simulink model "QueuingStrategies_513"  (R2019b)
settings: Solver=VariableStepAuto  StartTime=0.0  StopTime=1000  RelTol=1e-3  EnableMultiTasking=on
InitFcn:
  | a = randi(600);
  | rng(a)
undefined symbols (not defined in the file or in its folder): elapsedTime, entity, m, n, whichLine
libraries: simulink x1
settings Model: Creator=The MathWorks, Inc.  LastModifiedBy=thb
settings DataIOCC: ReturnWorkspaceOutputs=off
settings OptimizationCC: LifeSpan=inf
settings DebuggingCC: SFUnexpectedBacktrackingDiag=warning  SFNoUnconditionalDefaultTransitionDiag=warning  SFExecutionAtInitializationDiag=none  ArithmeticOperatorsInVariantConditions=warning
settings SFSimCC: SimUseLocalCustomCode=off  CustomCodeUndefinedFunction=UseInterfaceOnly
settings RTWCC: RTWUseLocalCustomCode=off
settings CodeAppCC: StateflowObjectComments=on
settings GRTTargetCC: TargetLangStandard=C89/C90 (ANSI)
settings ConfigComp: CovMetricSettings=dw  CovHtmlReporting=on  CovSaveCumulativeToWorkspaceVar=on  CovSaveSingleToWorkspaceVar=on  CovExternalEMLEnable=off

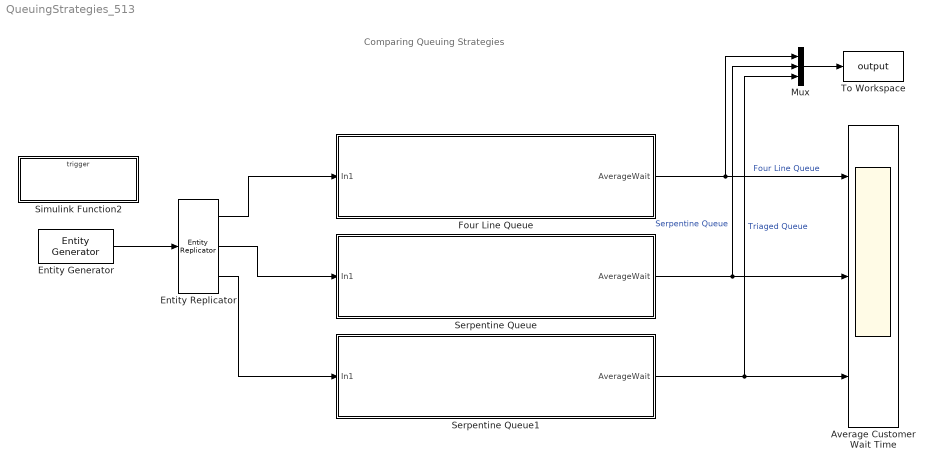
== system QueuingStrategies_513 ==
  note: Comparing Queuing Strategies
  "Average Customer Wait Time " : Scope  NumInputPorts=3
  Entity Generator : EntityGenerator  OutputPortMessageModes=m  TimeSource=MATLAB action  Period=.75  IntergenerationTimeAction=|  GenerateAction=|  AttributeName=ServiceTime|TimeStamp|QueuePath  AttributeInitialValue=0|0|0  EntityType=Structured  EntityTypeName=Customer
      IntergenerationTimeAction=|
      | % Exponential arrival process with rate 1
      | persistent rngInit;
      | if isempty(rngInit)
      |     seed = random_seed;
      |     rng(seed);
      |     rngInit = true;
      | end
      | 
      | 
      | mean = 1;
      | dt = -mean*log(1-rand());
      GenerateAction=|
      | % Exponential service process with rate 2
      | persistent rngInit;
      | if isempty(rngInit)
      |     seed = random_seed;
      |     rng(seed);
      |     rngInit = true;
      | end
      | 
      | mean = 2;
      | entity.ServiceTime = -mean*log(1-rand());
      | 
      | % Record time of generation so we can
      | % compute waiting time
      | entity.TimeStamp = stampEntity();
  Entity Replicator : EntityReplicator  InputPortMessageModes=m  OutputPortMessageModes=m,m,m  NumberReplicas=2
      settings: OutputPortMap=o0,o1,o2
  Four Line Queue : Subsystem
      mask Display: disp('Four Line Queue\n\nSeparate Queue for Each Cash Register');
  Mux : Mux  Inputs=3
  Serpentine Queue : Subsystem
      mask Display: disp('Serpentine Queue\n\nSingle Queue for all Cash Registers');
  Serpentine Queue1 : Subsystem
      mask Display: disp('Triaged Queue\n\n1 Fast Queue 1 Slow Queue');
  Simulink Function2 : Subsystem  TreatAsAtomicUnit=on
  To Workspace : ToWorkspace  VariableName=output  SampleTime=-1
  wires:
  Entity Generator/1 -> Entity Replicator/1
  Entity Replicator/1 -> Four Line Queue/1(In1)
  Entity Replicator/2 -> Serpentine Queue/1(In1)
  Entity Replicator/3 -> Serpentine Queue1/1(In1)
  Four Line Queue/1(AverageWait) -> Mux/1, "Average Customer Wait Time "/1  "Four Line Queue"
  Serpentine Queue/1(AverageWait) -> Mux/2, "Average Customer Wait Time "/2  "Serpentine Queue"
  Serpentine Queue1/1(AverageWait) -> Mux/3, "Average Customer Wait Time "/3  "Triaged Queue"
  Mux/1 -> To Workspace/1

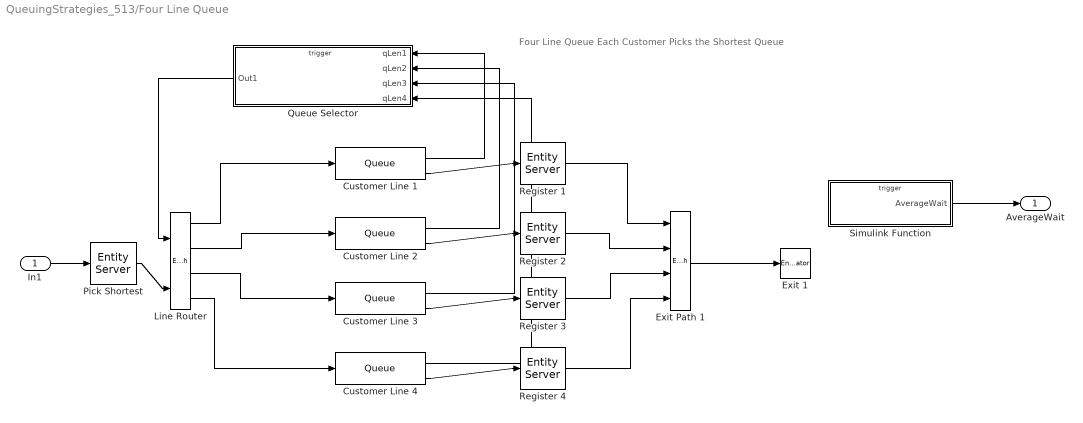
== system QueuingStrategies_513/Four Line Queue ==
  note: Four Line Queue
      | Each Customer Picks the Shortest Queue
  In1 : Inport
  Customer Line {1..4} (4 alike) : Queue  InputPortMessageModes=m  OutputPortMessageModes=n,m  Capacity=inf  NumberEntitiesInBlock=on
      settings: OutputPortMap=o1,o5
  Exit 1 : EntityTerminator  InputPortMessageModes=m  EntryAction=elapsedTime(entity.TimeStamp);
  Exit Path 1 : EntityInputSwitch  InputPortMessageModes=m,m,m,m  OutputPortMessageModes=m  NumberInputPorts=4
      settings: InputPortMap=u1,u2,u3,u4
  Line Router : EntityOutputSwitch  InputPortMessageModes=m,m  OutputPortMessageModes=m,m,m,m  NumberOutputPorts=4  SwitchingCriterion=From control port  SwitchAttributeName=QueuePath
      settings: InputPortMap=u0,u1  OutputPortMap=o0,o1,o2,o3
  Pick Shortest : EntityServer  InputPortMessageModes=m  OutputPortMessageModes=m  Capacity=1  ServiceTimeValue=0  EntryAction=|
      | % Entity will select the shortest queue
      | pickShortestQueue();
  Queue Selector : Subsystem  TreatAsAtomicUnit=on
  Register {1..4} (4 alike) : EntityServer  InputPortMessageModes=m  OutputPortMessageModes=m  Capacity=1  ServiceTimeSource=Attribute
  Simulink Function : Subsystem  TreatAsAtomicUnit=on
  AverageWait : Outport  VectorParamsAs1DForOutWhenUnconnected=off
  wires:
  Line Router/2 -> Customer Line 2/1
  Customer Line 2/1 -> Queue Selector/2(qLen2)
  Customer Line 3/2 -> Register 3/1
  Register 2/1 -> Exit Path 1/2
  Line Router/3 -> Customer Line 3/1
  Customer Line 1/2 -> Register 1/1
  Exit Path 1/1 -> Exit 1/1
  Customer Line 3/1 -> Queue Selector/3(qLen3)
  Customer Line 1/1 -> Queue Selector/1(qLen1)
  Register 4/1 -> Exit Path 1/4
  Register 1/1 -> Exit Path 1/1
  Customer Line 2/2 -> Register 2/1
  Register 3/1 -> Exit Path 1/3
  Queue Selector/1(Out1) -> Line Router/1
  Customer Line 4/2 -> Register 4/1
  In1/1 -> Pick Shortest/1
  Line Router/4 -> Customer Line 4/1
  Line Router/1 -> Customer Line 1/1
  Customer Line 4/1 -> Queue Selector/4(qLen4)
  Pick Shortest/1 -> Line Router/2
  Simulink Function/1(AverageWait) -> AverageWait/1

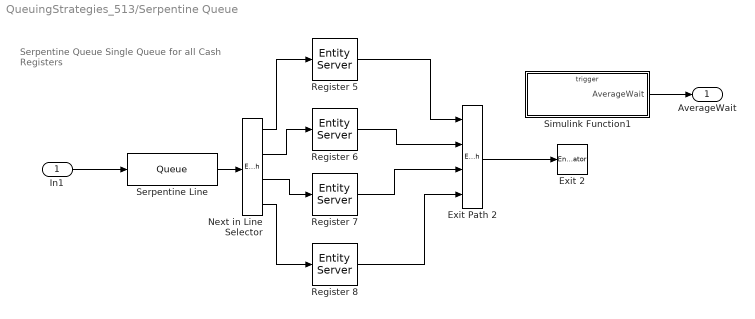
== system QueuingStrategies_513/Serpentine Queue ==
  note: Serpentine Queue
      | Single Queue for all Cash Registers
  In1 : Inport
  Exit 2 : EntityTerminator  InputPortMessageModes=m  EntryAction=elapsedTime(entity.TimeStamp);
  Exit Path 2 : EntityInputSwitch  InputPortMessageModes=m,m,m,m  OutputPortMessageModes=m  NumberInputPorts=4
      settings: InputPortMap=u1,u2,u3,u4
  Next in Line Selector : EntityOutputSwitch  InputPortMessageModes=m  OutputPortMessageModes=m,m,m,m  NumberOutputPorts=4  SwitchAttributeName=Attribute1
      settings: OutputPortMap=o0,o1,o2,o3
  Register {5..8} (4 alike) : EntityServer  InputPortMessageModes=m  OutputPortMessageModes=m  Capacity=1  ServiceTimeSource=Attribute
  Serpentine Line : Queue  InputPortMessageModes=m  OutputPortMessageModes=m  Capacity=inf
  Simulink Function1 : Subsystem  TreatAsAtomicUnit=on
  AverageWait : Outport  VectorParamsAs1DForOutWhenUnconnected=off
  wires:
  Next in Line Selector/2 -> Register 6/1
  Exit Path 2/1 -> Exit 2/1
  Serpentine Line/1 -> Next in Line Selector/1
  Next in Line Selector/4 -> Register 8/1
  In1/1 -> Serpentine Line/1
  Register 8/1 -> Exit Path 2/4
  Register 7/1 -> Exit Path 2/3
  Register 5/1 -> Exit Path 2/1
  Register 6/1 -> Exit Path 2/2
  Next in Line Selector/1 -> Register 5/1
  Next in Line Selector/3 -> Register 7/1
  Simulink Function1/1(AverageWait) -> AverageWait/1

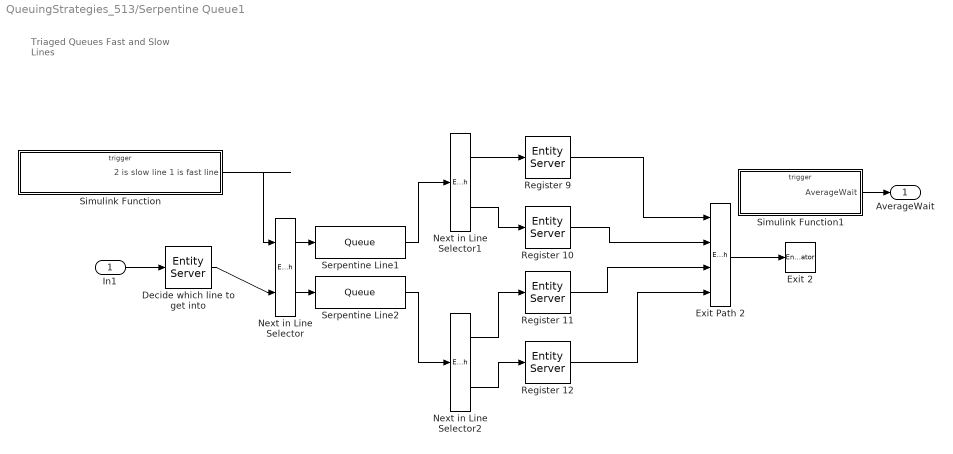
== system QueuingStrategies_513/Serpentine Queue1 ==
  note: Triaged Queues
      | Fast and Slow Lines
  In1 : Inport
  Decide which line to get into : EntityServer  InputPortMessageModes=m  OutputPortMessageModes=m  Capacity=1  ServiceTimeValue=0  ExitAction=whichLine(entity.ServiceTime)
  Exit 2 : EntityTerminator  InputPortMessageModes=m  EntryAction=elapsedTime(entity.TimeStamp);
  Exit Path 2 : EntityInputSwitch  InputPortMessageModes=m,m,m,m  OutputPortMessageModes=m  NumberInputPorts=4
      settings: InputPortMap=u1,u2,u3,u4
  Next in Line Selector : EntityOutputSwitch  InputPortMessageModes=m,m  OutputPortMessageModes=m,m  SwitchingCriterion=From control port  SwitchAttributeName=Attribute1
      settings: InputPortMap=u0,u1
  Next in Line Selector1 : EntityOutputSwitch  InputPortMessageModes=m  OutputPortMessageModes=m,m  SwitchAttributeName=Attribute1
  Next in Line Selector2 : EntityOutputSwitch  InputPortMessageModes=m  OutputPortMessageModes=m,m  SwitchAttributeName=Attribute1
  Register {9..12} (4 alike) : EntityServer  InputPortMessageModes=m  OutputPortMessageModes=m  Capacity=1  ServiceTimeSource=Attribute
  Serpentine Line1 : Queue  InputPortMessageModes=m  OutputPortMessageModes=m  Capacity=inf
  Serpentine Line2 : Queue  InputPortMessageModes=m  OutputPortMessageModes=m  Capacity=inf
  Simulink Function : Subsystem  TreatAsAtomicUnit=on
  Simulink Function1 : Subsystem  TreatAsAtomicUnit=on
  AverageWait : Outport  VectorParamsAs1DForOutWhenUnconnected=off
  wires:
  Register 10/1 -> Exit Path 2/2
  Register 9/1 -> Exit Path 2/1
  Register 11/1 -> Exit Path 2/3
  Register 12/1 -> Exit Path 2/4
  In1/1 -> Decide which line to get into/1
  Exit Path 2/1 -> Exit 2/1
  Simulink Function/1("2 is slow line 1 is fast line ") -> Next in Line Selector/1
  Next in Line Selector/1 -> Serpentine Line1/1
  Next in Line Selector/2 -> Serpentine Line2/1
  Next in Line Selector1/1 -> Register 9/1
  Simulink Function1/1(AverageWait) -> AverageWait/1
  Next in Line Selector1/2 -> Register 10/1
  Next in Line Selector2/1 -> Register 11/1
  Next in Line Selector2/2 -> Register 12/1
  Serpentine Line2/1 -> Next in Line Selector2/1
  Serpentine Line1/1 -> Next in Line Selector1/1
  Decide which line to get into/1 -> Next in Line Selector/2

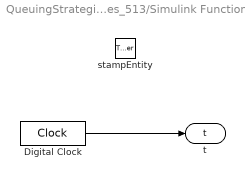
== system QueuingStrategies_513/Simulink Function2 ==
  stampEntity : TriggerPort  TriggerType=function-call  IsSimulinkFunction=on  FunctionName=stampEntity  VariantControl=Variant
  Digital Clock : DigitalClock  SampleTime=-1
  t : ArgOut  DisableCoverage=on  ArgumentName=t
  wires:
  Digital Clock/1 -> t/1

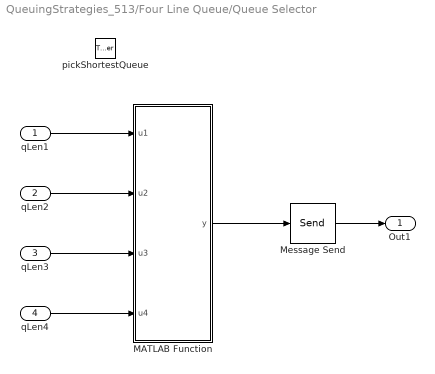
== system QueuingStrategies_513/Four Line Queue/Queue Selector ==
  qLen1 : Inport
  qLen2 : Inport  Port=2
  qLen3 : Inport  Port=3
  qLen4 : Inport  Port=4
  pickShortestQueue : TriggerPort  TriggerType=function-call  IsSimulinkFunction=on  FunctionName=pickShortestQueue  FunctionVisibility=scoped  VariantControl=Variant
  MATLAB Function : MATLAB Function  TreatAsAtomicUnit=on
  Message Send : Send  OutputPortMessageModes=m
  Out1 : Outport  VectorParamsAs1DForOutWhenUnconnected=off
  wires:
  qLen1/1 -> MATLAB Function/1(u1)
  qLen2/1 -> MATLAB Function/2(u2)
  qLen3/1 -> MATLAB Function/3(u3)
  qLen4/1 -> MATLAB Function/4(u4)
  MATLAB Function/1(y) -> Message Send/1
  Message Send/1 -> Out1/1

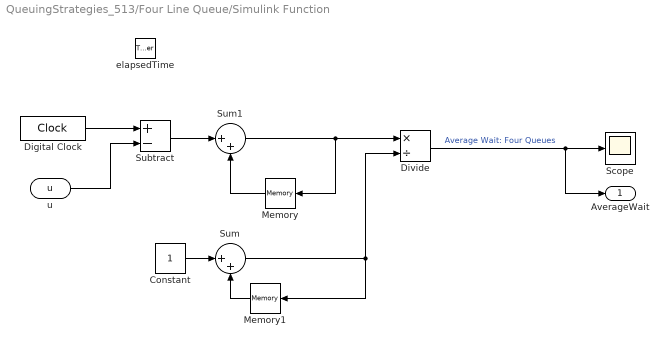
== system QueuingStrategies_513/Four Line Queue/Simulink Function ==
  elapsedTime : TriggerPort  TriggerType=function-call  IsSimulinkFunction=on  FunctionName=elapsedTime  FunctionVisibility=scoped  VariantControl=Variant
  Constant : Constant
  Digital Clock : DigitalClock  SampleTime=-1
  Divide : Product  Inputs=*/
  Memory : Memory  InheritSampleTime=on
  Memory1 : Memory  InheritSampleTime=on
  Scope : Scope
  Subtract : Sum  Inputs=+-
  Sum : Sum  Inputs=|++
  Sum1 : Sum  Inputs=|++
  u : ArgIn  DisableCoverage=on  ArgumentName=u
  AverageWait : Outport  VectorParamsAs1DForOutWhenUnconnected=off
  wires:
  Digital Clock/1 -> Subtract/1
  u/1 -> Subtract/2
  Subtract/1 -> Sum1/1
  Constant/1 -> Sum/1
  Memory1/1 -> Sum/2
  Sum/1 -> Memory1/1, Divide/2
  Divide/1 -> AverageWait/1, Scope/1  "Average Wait: Four Queues"
  Sum1/1 -> Memory/1, Divide/1
  Memory/1 -> Sum1/2

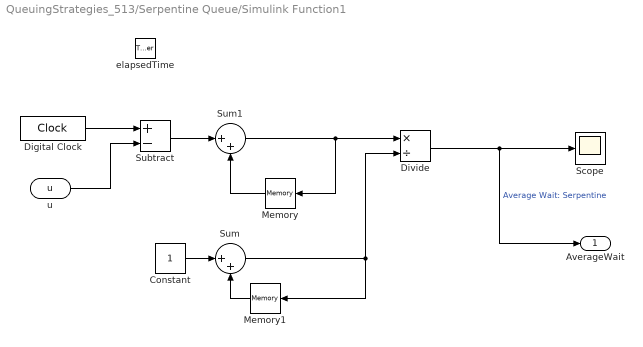
== system QueuingStrategies_513/Serpentine Queue/Simulink Function1 ==
  elapsedTime : TriggerPort  TriggerType=function-call  IsSimulinkFunction=on  FunctionName=elapsedTime  FunctionVisibility=scoped  VariantControl=Variant
  Constant : Constant
  Digital Clock : DigitalClock  SampleTime=-1
  Divide : Product  Inputs=*/
  Memory : Memory  InheritSampleTime=on
  Memory1 : Memory  InheritSampleTime=on
  Scope : Scope
  Subtract : Sum  Inputs=+-
  Sum : Sum  Inputs=|++
  Sum1 : Sum  Inputs=|++
  u : ArgIn  DisableCoverage=on  ArgumentName=u
  AverageWait : Outport  VectorParamsAs1DForOutWhenUnconnected=off
  wires:
  Memory/1 -> Sum1/2
  Sum1/1 -> Divide/1, Memory/1
  Divide/1 -> AverageWait/1, Scope/1  "Average Wait: Serpentine"
  Sum/1 -> Divide/2, Memory1/1
  Memory1/1 -> Sum/2
  Constant/1 -> Sum/1
  Subtract/1 -> Sum1/1
  u/1 -> Subtract/2
  Digital Clock/1 -> Subtract/1

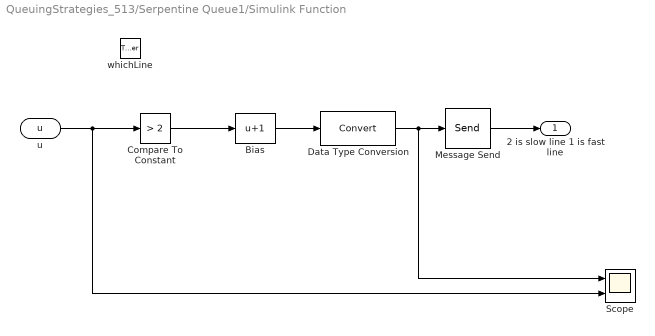
== system QueuingStrategies_513/Serpentine Queue1/Simulink Function ==
  whichLine : TriggerPort  TriggerType=function-call  IsSimulinkFunction=on  FunctionName=whichLine  FunctionVisibility=scoped  VariantControl=(inherit)
  Bias : Bias  Bias=1
  Compare To Constant : simulink/Logic and Bit Operations/Compare To Constant  relop=>  const=2  OutDataTypeStr=uint8
  Data Type Conversion : DataTypeConversion
  Message Send : Send  OutputPortMessageModes=m
  Scope : Scope  NumInputPorts=2
  u : ArgIn  DisableCoverage=on  ArgumentName=u
  "2 is slow line 1 is fast line " : Outport  VectorParamsAs1DForOutWhenUnconnected=off
  wires:
  u/1 -> Scope/2, Compare To Constant/1
  Compare To Constant/1 -> Bias/1
  Bias/1 -> Data Type Conversion/1
  Data Type Conversion/1 -> Scope/1, Message Send/1
  Message Send/1 -> "2 is slow line 1 is fast line "/1

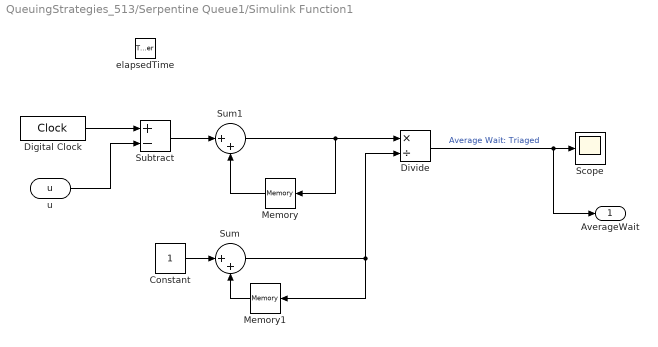
== system QueuingStrategies_513/Serpentine Queue1/Simulink Function1 ==
  elapsedTime : TriggerPort  TriggerType=function-call  IsSimulinkFunction=on  FunctionName=elapsedTime  FunctionVisibility=scoped  VariantControl=Variant
  Constant : Constant
  Digital Clock : DigitalClock  SampleTime=-1
  Divide : Product  Inputs=*/
  Memory : Memory  InheritSampleTime=on
  Memory1 : Memory  InheritSampleTime=on
  Scope : Scope
  Subtract : Sum  Inputs=+-
  Sum : Sum  Inputs=|++
  Sum1 : Sum  Inputs=|++
  u : ArgIn  DisableCoverage=on  ArgumentName=u
  AverageWait : Outport  VectorParamsAs1DForOutWhenUnconnected=off
  wires:
  Digital Clock/1 -> Subtract/1
  u/1 -> Subtract/2
  Subtract/1 -> Sum1/1
  Constant/1 -> Sum/1
  Memory1/1 -> Sum/2
  Sum/1 -> Memory1/1, Divide/2
  Divide/1 -> AverageWait/1, Scope/1  "Average Wait: Triaged"
  Sum1/1 -> Memory/1, Divide/1
  Memory/1 -> Sum1/2

== matlab function QueuingStrategies_513/Four Line Queue/Queue Selector/MATLAB Function ==
  data: u1 input; y output; u2 input; u3 input; u4 input
function y = fcn(u1, u2, u3, u4)
%#codegen

% Identify which input index is the smallest
[a,y] = min([u1 u2 u3 u4]);
